simulink model "Ex2_Sim"  (R2021b)
settings: Solver=VariableStepAuto  StartTime=0.0  StopTime=10.0  RelTol=1e-3

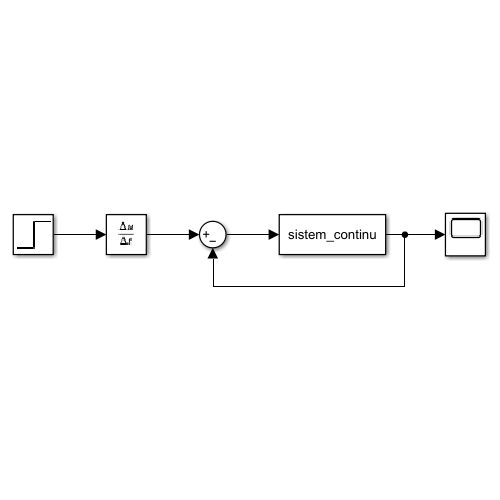
[thumbnail: Simulink's stored preview of the top-level diagram]
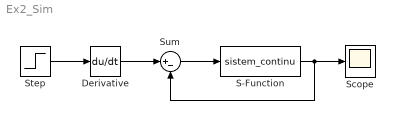
== system Ex2_Sim ==
  Derivative : Derivative
  S-Function : S-Function  FunctionName=sistem_continu  Parameters=[-3 -6; 1 0], [1;0], [0 6],[1]  SFunctionDeploymentMode=off  EnableBusSupport=off
  Scope : Scope
  Step : Step  SampleTime=0
  Sum : Sum  Inputs=|+-
  wires:
  Sum/1 -> S-Function/1
  Step/1 -> Derivative/1
  S-Function/1 -> Sum/2, Scope/1
  Derivative/1 -> Sum/1
